simulink model "gate_V32_2016a_Sim"  (R2016a)
settings: Solver=FixedStepDiscrete  StartTime=0.0  StopTime=120  FixedStep=0.001  RelTol=1e-3
undefined symbols (not defined in the file): CLOSE_CHAR, CLOSE_SIDE_VALUE, CLOSED, CLOSING, CURRENT_STABLE_TIMER, CURRENT_THRESH, INIT, MOVING_TIMER, NO_PASS_ASSIG, OPEN, OPEN_CHAR, OPEN_SIDE_VALUE, OPEN_TIMEOUT, OPENING, OPENING_ACTIVE, PASS_ASSIGNED, PASS_INCOMPLETE, PASS_TIMEOUT, PASSWORD_VERIFIED, STABLE_TIMER_VALUE, TIMEOUT, WRONG_PASSWORD
(part 1 of 2)
settings Model: ExtModeTrigDuration=2  Creator=omaro  LastModifiedBy=oelkawok
settings DataIOCC: SaveFormat=StructureWithTime
settings OptimizationCC: DefaultParameterBehavior=Inlined  StateBitsets=on  DataBitsets=on  LifeSpan=1  MaxStackSize=64
settings DebuggingCC: ConsistencyChecking=error  ArrayBoundsChecking=error  SignalInfNanChecking=error  SignalRangeChecking=error  ReadBeforeWriteMsg=EnableAllAsError  WriteAfterWriteMsg=EnableAllAsError  WriteAfterReadMsg=EnableAllAsError  AlgebraicLoopMsg=error  ArtificialAlgebraicLoopMsg=error  BlockPriorityViolationMsg=error  MinStepSizeMsg=error  CheckMatrixSingularityMsg=error  ParameterUnderflowMsg=error  ParameterPrecisionLossMsg=error  UnderSpecifiedDataTypeMsg=warning  UnnecessaryDatatypeConvMsg=warning  VectorMatrixConversionMsg=error  SignalLabelMismatchMsg=error  UnconnectedInputMsg=error  UnconnectedOutputMsg=error  UnconnectedLineMsg=error  SFcnCompatibilityMsg=error  UniqueDataStoreMsg=error  BusObjectLabelMismatch=error  RootOutportRequireBusObject=error  ModelReferenceIOMsg=error  ModelReferenceVersionMismatchMessage=error  ModelReferenceIOMismatchMessage=error  ModelReferenceDataLoggingMessage=error  StrictBusMsg=ErrorOnBusTreatedAsVector  SFUnusedDataAndEventsDiag=error  SFUnexpectedBacktrackingDiag=error  SFInvalidInputDataAccessInChartInitDiag=error  SFNoUnconditionalDefaultTransitionDiag=error  SFTransitionOutsideNaturalParentDiag=error  SFUndirectedBroadcastEventsDiag=error  SFTransitionActionBeforeConditionDiag=error  SFOutputUsedAsStateInMooreChartDiag=warning
settings HardwareCC: ProdLongLongMode=on
settings SFSimCC: SimCustomHeaderCode=|
  | //#include "C:\Users\omaro\Desktop\Gate_Model\Arduino\Arduino.h"
  | //#include "Keypad\Keypad.h"
settings RTWCC: SystemTargetFile=ert.tlc  TemplateMakefile=ert_default_tmf  GenerateReport=on  RTWUseSimCustomCode=on  Toolchain=Arduino AVR v1.6.1  BuildConfiguration=Faster Runs  LaunchReport=on
settings RTWCC: CustomHeaderCode=|
  | //#include "C:\Users\omaro\Desktop\Gate_Model\Arduino\Arduino.h"
  | //#include "Keypad\Keypad.h"
settings CodeAppCC: ForceParamTrailComments=on  OperatorAnnotations=on  MATLABSourceComments=on
settings ERTTargetCC: ERTCustomFileBanners=off  SupportContinuousTime=on  SupportNonInlinedSFcns=on  SupportVariableSizeSignals=on  ModelStepFunctionPrototypeControlCompliant=off  RootIOFormat=Structure reference  ERTCustomFileTemplate=example_file_process.tlc

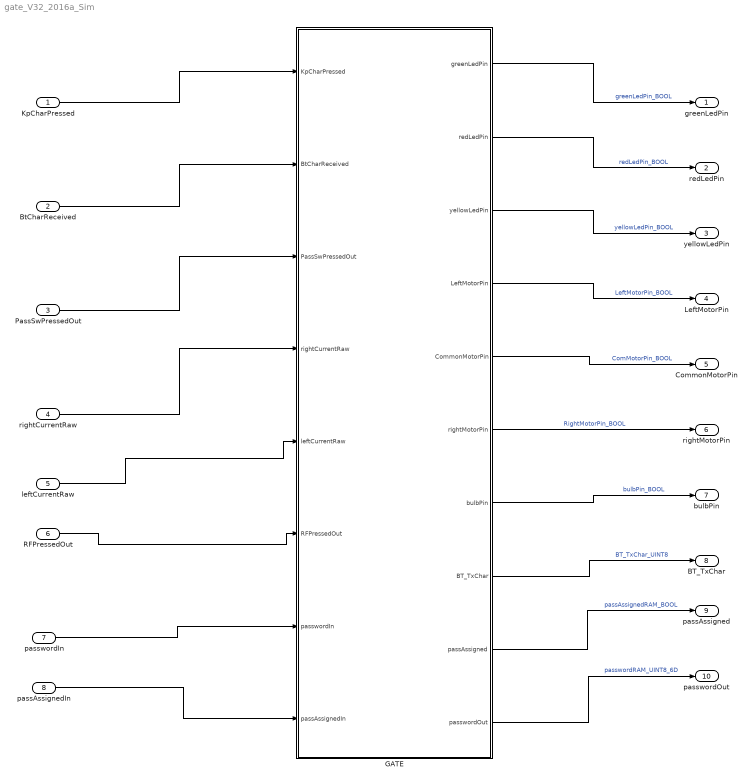
== system gate_V32_2016a_Sim ==
  "KpCharPressed " : Inport
  "BtCharReceived " : Inport  Port=2
  "PassSwPressedOut " : Inport  Port=3
  rightCurrentRaw : Inport  Port=4
  leftCurrentRaw : Inport  Port=5
  RFPressedOut : Inport  Port=6
  passwordIn : Inport  Port=7
  passAssignedIn : Inport  Port=8
  GATE : Subsystem  Variant=on  VariantControl=Variant1  OverrideUsingVariant=VariantB
  " greenLedPin" : Outport
  " redLedPin" : Outport  Port=2
  " yellowLedPin" : Outport  Port=3
  " LeftMotorPin" : Outport  Port=4
  " CommonMotorPin" : Outport  Port=5
  " rightMotorPin" : Outport  Port=6
  " bulbPin" : Outport  Port=7
  " BT_TxChar" : Outport  Port=8
  passAssigned : Outport  Port=9
  passwordOut : Outport  Port=10
  wires:
  passwordIn/1 -> GATE/7(passwordIn)
  "KpCharPressed "/1 -> GATE/1("KpCharPressed ")
  passAssignedIn/1 -> GATE/8(passAssignedIn)
  "BtCharReceived "/1 -> GATE/2("BtCharReceived ")
  leftCurrentRaw/1 -> GATE/5(leftCurrentRaw)
  "PassSwPressedOut "/1 -> GATE/3("PassSwPressedOut ")
  rightCurrentRaw/1 -> GATE/4(rightCurrentRaw)
  RFPressedOut/1 -> GATE/6(RFPressedOut)
  GATE/6(" rightMotorPin") -> " rightMotorPin"/1  "RightMotorPin_BOOL"
  GATE/5(" CommonMotorPin") -> " CommonMotorPin"/1  "ComMotorPin_BOOL"
  GATE/7(" bulbPin") -> " bulbPin"/1  "bulbPin_BOOL"
  GATE/4(" LeftMotorPin") -> " LeftMotorPin"/1  "LeftMotorPin_BOOL"
  GATE/8(" BT_TxChar") -> " BT_TxChar"/1  "BT_TxChar_UINT8"
  GATE/3(" yellowLedPin") -> " yellowLedPin"/1  "yellowLedPin_BOOL"
  GATE/2(" redLedPin") -> " redLedPin"/1  "redLedPin_BOOL"
  GATE/1(" greenLedPin") -> " greenLedPin"/1  "greenLedPin_BOOL"
  GATE/9(passAssigned) -> passAssigned/1  "passAssignedRAM_BOOL"
  GATE/10(passwordOut) -> passwordOut/1  "passwordRAM_UINT8_6D"

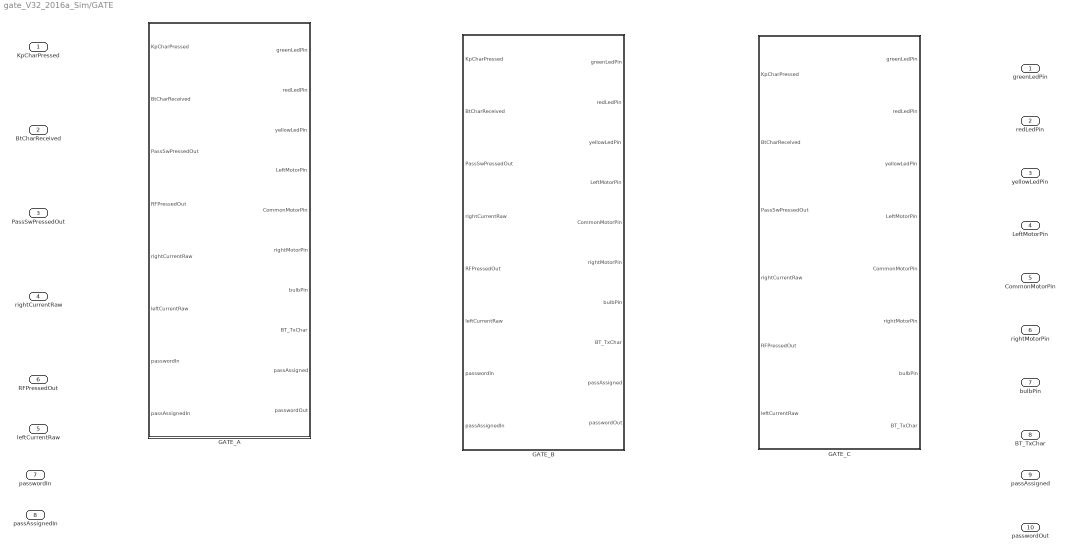
== system gate_V32_2016a_Sim/GATE ==
  "KpCharPressed " : Inport
  "BtCharReceived " : Inport  Port=2
  "PassSwPressedOut " : Inport  Port=3
  rightCurrentRaw : Inport  Port=4
  leftCurrentRaw : Inport  Port=5
  RFPressedOut : Inport  Port=6
  passwordIn : Inport  Port=7
  passAssignedIn : Inport  Port=8
  GATE_A : Subsystem  VariantControl=VariantA
  GATE_B : Subsystem  VariantControl=VariantB
  GATE_C : Subsystem  VariantControl=VariantC
  " greenLedPin" : Outport
  " redLedPin" : Outport  Port=2
  " yellowLedPin" : Outport  Port=3
  " LeftMotorPin" : Outport  Port=4
  " CommonMotorPin" : Outport  Port=5
  " rightMotorPin" : Outport  Port=6
  " bulbPin" : Outport  Port=7
  " BT_TxChar" : Outport  Port=8
  passAssigned : Outport  Port=9
  passwordOut : Outport  Port=10

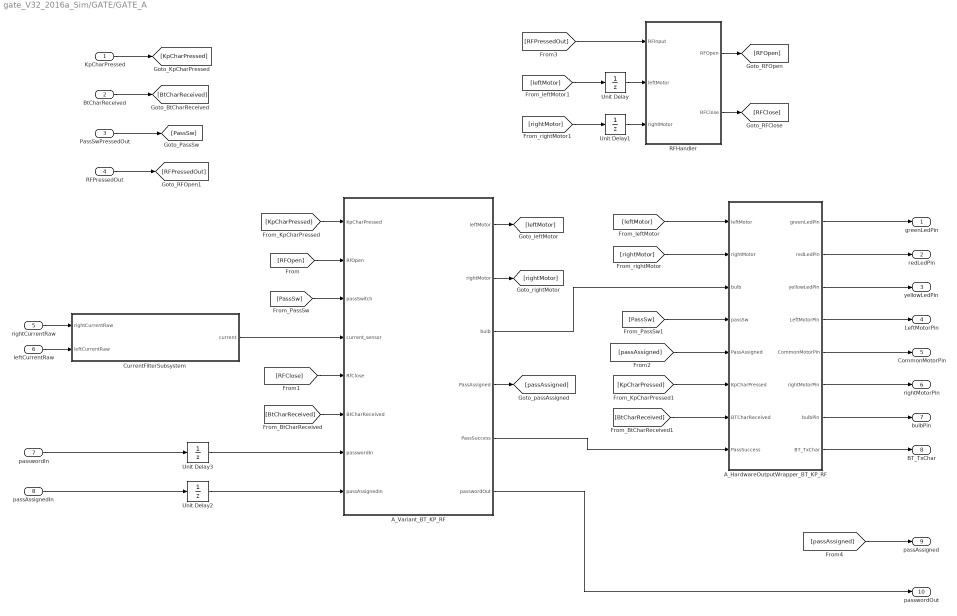
== system gate_V32_2016a_Sim/GATE/GATE_A ==
  KpCharPressed : Inport
  BtCharReceived : Inport  Port=2
  PassSwPressedOut : Inport  Port=3
  RFPressedOut : Inport  Port=4
  rightCurrentRaw : Inport  Port=5
  leftCurrentRaw : Inport  Port=6
  passwordIn : Inport  Port=7
  passAssignedIn : Inport  Port=8
  A_HardwareOutputWrapper_BT_KP_RF : Subsystem  VariantControl=Variant1
  A_Variant_BT_KP_RF : Subsystem  VariantControl=Variant
  CurrentFilterSubsystem : Subsystem
  RFHandler : Subsystem
  Unit Delay{,1..3} (4 alike) : UnitDelay  SampleTime=-1
  greenLedPin : Outport
  redLedPin : Outport  Port=2
  yellowLedPin : Outport  Port=3
  LeftMotorPin : Outport  Port=4
  CommonMotorPin : Outport  Port=5
  rightMotorPin : Outport  Port=6
  bulbPin : Outport  Port=7
  BT_TxChar : Outport  Port=8
  passAssigned : Outport  Port=9
  passwordOut : Outport  Port=10
  wires:
  RFHandler/1(RFOpen) -> [RFOpen]
  RFHandler/2(RFClose) -> [RFClose]
  [RFPressedOut] -> RFHandler/1(RFInput)
  RFPressedOut/1 -> [RFPressedOut]
  PassSwPressedOut/1 -> [PassSw]
  [leftMotor] -> Unit Delay/1
  Unit Delay/1 -> RFHandler/2(leftMotor)
  [rightMotor] -> Unit Delay1/1
  Unit Delay1/1 -> RFHandler/3(rightMotor)
  BtCharReceived/1 -> [BtCharReceived]
  KpCharPressed/1 -> [KpCharPressed]
  [RFOpen] -> A_Variant_BT_KP_RF/2(RfOpen)
  [PassSw] -> A_Variant_BT_KP_RF/3(passSwitch)
  [RFClose] -> A_Variant_BT_KP_RF/5(RfClose)
  [BtCharReceived] -> A_Variant_BT_KP_RF/6(BtCharReceived)
  A_Variant_BT_KP_RF/1(leftMotor) -> [leftMotor]
  A_Variant_BT_KP_RF/2(rightMotor) -> [rightMotor]
  [KpCharPressed] -> A_Variant_BT_KP_RF/1(KpCharPressed)
  [leftMotor] -> A_HardwareOutputWrapper_BT_KP_RF/1(leftMotor)
  [rightMotor] -> A_HardwareOutputWrapper_BT_KP_RF/2(rightMotor)
  A_Variant_BT_KP_RF/3(bulb) -> A_HardwareOutputWrapper_BT_KP_RF/3(bulb)
  [PassSw] -> A_HardwareOutputWrapper_BT_KP_RF/4(passSw)
  [KpCharPressed] -> A_HardwareOutputWrapper_BT_KP_RF/6(KpCharPressed)
  [BtCharReceived] -> A_HardwareOutputWrapper_BT_KP_RF/7(BTCharReceived)
  A_HardwareOutputWrapper_BT_KP_RF/1(greenLedPin) -> greenLedPin/1
  A_HardwareOutputWrapper_BT_KP_RF/2(redLedPin) -> redLedPin/1
  A_HardwareOutputWrapper_BT_KP_RF/3(yellowLedPin) -> yellowLedPin/1
  A_HardwareOutputWrapper_BT_KP_RF/4(LeftMotorPin) -> LeftMotorPin/1
  A_HardwareOutputWrapper_BT_KP_RF/5(CommonMotorPin) -> CommonMotorPin/1
  A_HardwareOutputWrapper_BT_KP_RF/6(rightMotorPin) -> rightMotorPin/1
  A_HardwareOutputWrapper_BT_KP_RF/7(bulbPin) -> bulbPin/1
  A_HardwareOutputWrapper_BT_KP_RF/8(BT_TxChar) -> BT_TxChar/1
  A_Variant_BT_KP_RF/4(PassAssigned) -> [passAssigned]
  [passAssigned] -> A_HardwareOutputWrapper_BT_KP_RF/5(PassAssigned)
  Unit Delay2/1 -> A_Variant_BT_KP_RF/8(passAssignedIn)
  Unit Delay3/1 -> A_Variant_BT_KP_RF/7(passwordIn)
  A_Variant_BT_KP_RF/5(PassSuccess) -> A_HardwareOutputWrapper_BT_KP_RF/8(PassSuccess)
  CurrentFilterSubsystem/1(current) -> A_Variant_BT_KP_RF/4(current_sensor)
  rightCurrentRaw/1 -> CurrentFilterSubsystem/1(rightCurrentRaw)
  leftCurrentRaw/1 -> CurrentFilterSubsystem/2(leftCurrentRaw)
  passAssignedIn/1 -> Unit Delay2/1
  passwordIn/1 -> Unit Delay3/1
  A_Variant_BT_KP_RF/6(passwordOut) -> passwordOut/1
  [passAssigned] -> passAssigned/1

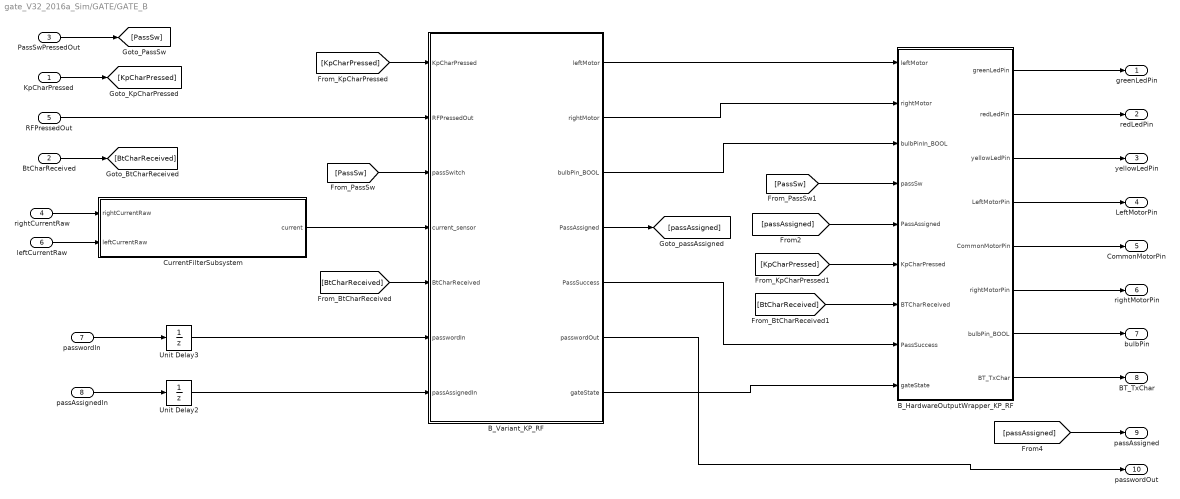
== system gate_V32_2016a_Sim/GATE/GATE_B ==
  KpCharPressed : Inport
  BtCharReceived : Inport  Port=2
  PassSwPressedOut : Inport  Port=3
  rightCurrentRaw : Inport  Port=4
  RFPressedOut : Inport  Port=5
  leftCurrentRaw : Inport  Port=6
  passwordIn : Inport  Port=7
  passAssignedIn : Inport  Port=8
  B_HardwareOutputWrapper_KP_RF : Subsystem  VariantControl=Variant2
  B_Variant_KP_RF : Subsystem  VariantControl=Variant2
  CurrentFilterSubsystem : Subsystem
  Unit Delay2 : UnitDelay  SampleTime=-1
  Unit Delay3 : UnitDelay  SampleTime=-1
  greenLedPin : Outport
  redLedPin : Outport  Port=2
  yellowLedPin : Outport  Port=3
  LeftMotorPin : Outport  Port=4
  CommonMotorPin : Outport  Port=5
  rightMotorPin : Outport  Port=6
  bulbPin : Outport  Port=7
  BT_TxChar : Outport  Port=8
  passAssigned : Outport  Port=9
  passwordOut : Outport  Port=10
  wires:
  CurrentFilterSubsystem/1(current) -> B_Variant_KP_RF/4(current_sensor)
  B_Variant_KP_RF/5(PassSuccess) -> B_HardwareOutputWrapper_KP_RF/8(PassSuccess)
  Unit Delay3/1 -> B_Variant_KP_RF/6(passwordIn)
  Unit Delay2/1 -> B_Variant_KP_RF/7(passAssignedIn)
  B_Variant_KP_RF/6(passwordOut) -> passwordOut/1
  [passAssigned] -> B_HardwareOutputWrapper_KP_RF/5(PassAssigned)
  B_Variant_KP_RF/4(PassAssigned) -> [passAssigned]
  B_HardwareOutputWrapper_KP_RF/8(BT_TxChar) -> BT_TxChar/1
  B_HardwareOutputWrapper_KP_RF/7(bulbPin_BOOL) -> bulbPin/1
  B_HardwareOutputWrapper_KP_RF/6(rightMotorPin) -> rightMotorPin/1
  B_HardwareOutputWrapper_KP_RF/5(CommonMotorPin) -> CommonMotorPin/1
  B_HardwareOutputWrapper_KP_RF/4(LeftMotorPin) -> LeftMotorPin/1
  B_HardwareOutputWrapper_KP_RF/3(yellowLedPin) -> yellowLedPin/1
  B_HardwareOutputWrapper_KP_RF/2(redLedPin) -> redLedPin/1
  B_HardwareOutputWrapper_KP_RF/1(greenLedPin) -> greenLedPin/1
  [BtCharReceived] -> B_HardwareOutputWrapper_KP_RF/7(BTCharReceived)
  [KpCharPressed] -> B_HardwareOutputWrapper_KP_RF/6(KpCharPressed)
  [PassSw] -> B_HardwareOutputWrapper_KP_RF/4(passSw)
  B_Variant_KP_RF/3(bulbPin_BOOL) -> B_HardwareOutputWrapper_KP_RF/3(bulbPinIn_BOOL)
  B_Variant_KP_RF/1(leftMotor) -> B_HardwareOutputWrapper_KP_RF/1(leftMotor)
  [KpCharPressed] -> B_Variant_KP_RF/1(KpCharPressed)
  [BtCharReceived] -> B_Variant_KP_RF/5(BtCharReceived)
  rightCurrentRaw/1 -> CurrentFilterSubsystem/1(rightCurrentRaw)
  [PassSw] -> B_Variant_KP_RF/3(passSwitch)
  RFPressedOut/1 -> B_Variant_KP_RF/2(RFPressedOut)
  KpCharPressed/1 -> [KpCharPressed]
  BtCharReceived/1 -> [BtCharReceived]
  PassSwPressedOut/1 -> [PassSw]
  leftCurrentRaw/1 -> CurrentFilterSubsystem/2(leftCurrentRaw)
  [passAssigned] -> passAssigned/1
  passAssignedIn/1 -> Unit Delay2/1
  passwordIn/1 -> Unit Delay3/1
  B_Variant_KP_RF/2(rightMotor) -> B_HardwareOutputWrapper_KP_RF/2(rightMotor)
  B_Variant_KP_RF/7(gateState) -> B_HardwareOutputWrapper_KP_RF/9(gateState)

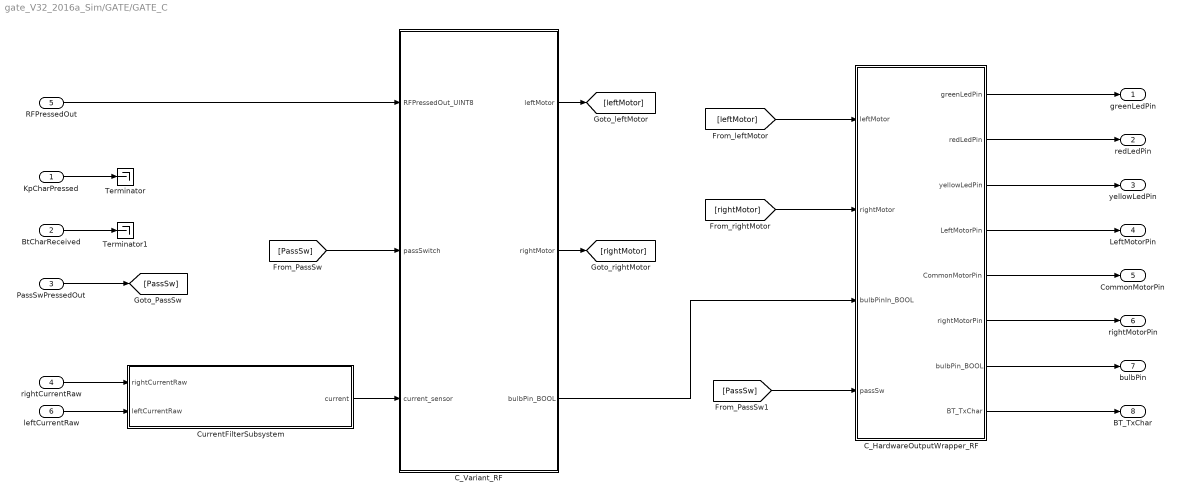
== system gate_V32_2016a_Sim/GATE/GATE_C ==
  KpCharPressed : Inport
  BtCharReceived : Inport  Port=2
  PassSwPressedOut : Inport  Port=3
  rightCurrentRaw : Inport  Port=4
  RFPressedOut : Inport  Port=5
  leftCurrentRaw : Inport  Port=6
  C_HardwareOutputWrapper_RF : Subsystem  VariantControl=Variant3
  C_Variant_RF : Subsystem  VariantControl=Variant3
  CurrentFilterSubsystem : Subsystem
  Terminator : Terminator
  Terminator1 : Terminator
  greenLedPin : Outport
  redLedPin : Outport  Port=2
  yellowLedPin : Outport  Port=3
  LeftMotorPin : Outport  Port=4
  CommonMotorPin : Outport  Port=5
  rightMotorPin : Outport  Port=6
  bulbPin : Outport  Port=7
  BT_TxChar : Outport  Port=8
  wires:
  PassSwPressedOut/1 -> [PassSw]
  BtCharReceived/1 -> Terminator1/1
  KpCharPressed/1 -> Terminator/1
  [PassSw] -> C_Variant_RF/2(passSwitch)
  rightCurrentRaw/1 -> CurrentFilterSubsystem/1(rightCurrentRaw)
  C_Variant_RF/1(leftMotor) -> [leftMotor]
  C_Variant_RF/2(rightMotor) -> [rightMotor]
  [leftMotor] -> C_HardwareOutputWrapper_RF/1(leftMotor)
  [rightMotor] -> C_HardwareOutputWrapper_RF/2(rightMotor)
  C_Variant_RF/3(bulbPin_BOOL) -> C_HardwareOutputWrapper_RF/3(bulbPinIn_BOOL)
  [PassSw] -> C_HardwareOutputWrapper_RF/4(passSw)
  C_HardwareOutputWrapper_RF/1(greenLedPin) -> greenLedPin/1
  C_HardwareOutputWrapper_RF/2(redLedPin) -> redLedPin/1
  C_HardwareOutputWrapper_RF/3(yellowLedPin) -> yellowLedPin/1
  C_HardwareOutputWrapper_RF/4(LeftMotorPin) -> LeftMotorPin/1
  C_HardwareOutputWrapper_RF/5(CommonMotorPin) -> CommonMotorPin/1
  C_HardwareOutputWrapper_RF/6(rightMotorPin) -> rightMotorPin/1
  C_HardwareOutputWrapper_RF/7(bulbPin_BOOL) -> bulbPin/1
  C_HardwareOutputWrapper_RF/8(BT_TxChar) -> BT_TxChar/1
  CurrentFilterSubsystem/1(current) -> C_Variant_RF/3(current_sensor)
  leftCurrentRaw/1 -> CurrentFilterSubsystem/2(leftCurrentRaw)
  RFPressedOut/1 -> C_Variant_RF/1(RFPressedOut_UINT8)

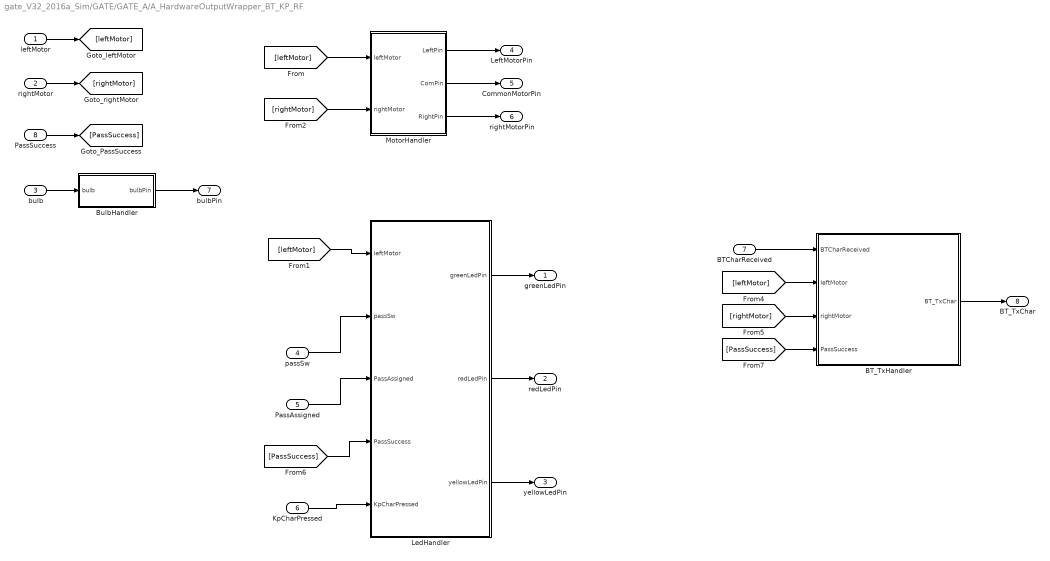
== system gate_V32_2016a_Sim/GATE/GATE_A/A_HardwareOutputWrapper_BT_KP_RF ==
  leftMotor : Inport
  rightMotor : Inport  Port=2
  bulb : Inport  Port=3
  passSw : Inport  Port=4
  PassAssigned : Inport  Port=5
  KpCharPressed : Inport  Port=6
  BTCharReceived : Inport  Port=7
  PassSuccess : Inport  Port=8
  BT_TxHandler : Subsystem
  BulbHandler : Subsystem
  LedHandler : Subsystem
  MotorHandler : Subsystem
  greenLedPin : Outport
  redLedPin : Outport  Port=2
  yellowLedPin : Outport  Port=3
  LeftMotorPin : Outport  Port=4
  CommonMotorPin : Outport  Port=5
  rightMotorPin : Outport  Port=6
  bulbPin : Outport  Port=7
  BT_TxChar : Outport  Port=8
  wires:
  [leftMotor] -> MotorHandler/1(leftMotor)
  [rightMotor] -> MotorHandler/2(rightMotor)
  bulb/1 -> BulbHandler/1(bulb)
  LedHandler/1(greenLedPin) -> greenLedPin/1
  LedHandler/2(redLedPin) -> redLedPin/1
  LedHandler/3(yellowLedPin) -> yellowLedPin/1
  MotorHandler/1(LeftPin) -> LeftMotorPin/1
  MotorHandler/2(ComPin) -> CommonMotorPin/1
  MotorHandler/3(RightPin) -> rightMotorPin/1
  BulbHandler/1(bulbPin) -> bulbPin/1
  leftMotor/1 -> [leftMotor]
  [leftMotor] -> LedHandler/1(leftMotor)
  rightMotor/1 -> [rightMotor]
  passSw/1 -> LedHandler/2(passSw)
  PassAssigned/1 -> LedHandler/3(PassAssigned)
  [PassSuccess] -> LedHandler/4(PassSuccess)
  KpCharPressed/1 -> LedHandler/5(KpCharPressed)
  [leftMotor] -> BT_TxHandler/2(leftMotor)
  BTCharReceived/1 -> BT_TxHandler/1(BTCharReceived)
  [rightMotor] -> BT_TxHandler/3(rightMotor)
  PassSuccess/1 -> [PassSuccess]
  [PassSuccess] -> BT_TxHandler/4(PassSuccess)
  BT_TxHandler/1(BT_TxChar) -> BT_TxChar/1

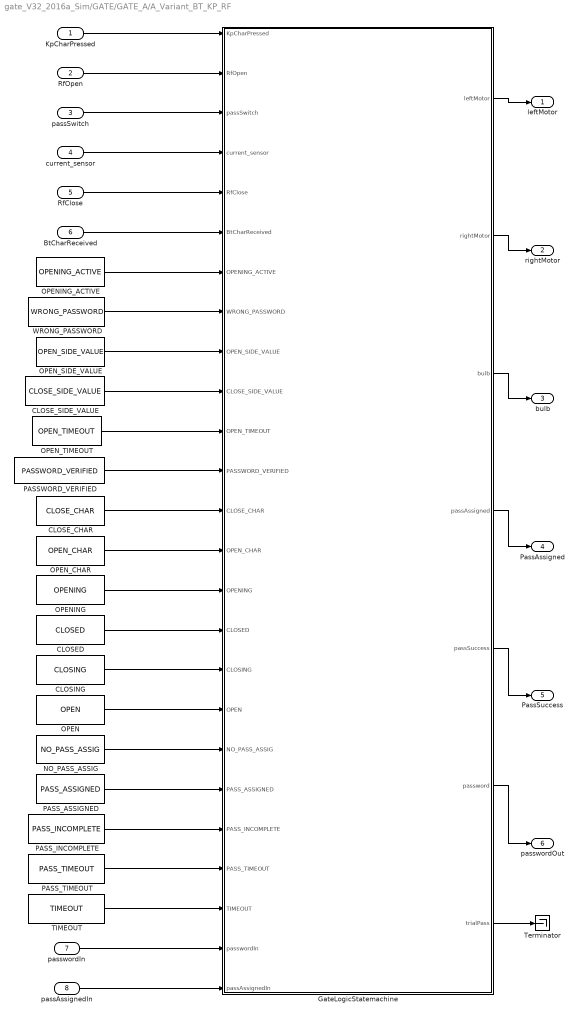
== system gate_V32_2016a_Sim/GATE/GATE_A/A_Variant_BT_KP_RF ==
  KpCharPressed : Inport
  RfOpen : Inport  Port=2
  passSwitch : Inport  Port=3
  current_sensor : Inport  Port=4
  RfClose : Inport  Port=5
  BtCharReceived : Inport  Port=6
  passwordIn : Inport  Port=7
  passAssignedIn : Inport  Port=8
  CLOSED : Constant  Value=CLOSED  SampleTime=-1
  CLOSE_CHAR : Constant  Value=CLOSE_CHAR  SampleTime=-1
  CLOSE_SIDE_VALUE : Constant  Value=CLOSE_SIDE_VALUE  SampleTime=-1
  CLOSING : Constant  Value=CLOSING  SampleTime=-1
  GateLogicStatemachine : Stateflow chart  TreatAsAtomicUnit=on
  NO_PASS_ASSIG : Constant  Value=NO_PASS_ASSIG  SampleTime=-1
  OPEN : Constant  Value=OPEN  SampleTime=-1
  OPENING : Constant  Value=OPENING  SampleTime=-1
  OPENING_ACTIVE : Constant  Value=OPENING_ACTIVE  SampleTime=-1
  OPEN_CHAR : Constant  Value=OPEN_CHAR  SampleTime=-1
  OPEN_SIDE_VALUE : Constant  Value=OPEN_SIDE_VALUE  SampleTime=-1
  OPEN_TIMEOUT : Constant  Value=OPEN_TIMEOUT  SampleTime=-1
  PASSWORD_VERIFIED : Constant  Value=PASSWORD_VERIFIED  SampleTime=-1
  PASS_ASSIGNED : Constant  Value=PASS_ASSIGNED  SampleTime=-1
  PASS_INCOMPLETE : Constant  Value=PASS_INCOMPLETE  SampleTime=-1
  PASS_TIMEOUT : Constant  Value=PASS_TIMEOUT  SampleTime=-1
  TIMEOUT : Constant  Value=TIMEOUT  SampleTime=-1
  Terminator : Terminator
  WRONG_PASSWORD : Constant  Value=WRONG_PASSWORD  SampleTime=-1
  leftMotor : Outport
  rightMotor : Outport  Port=2
  bulb : Outport  Port=3
  PassAssigned : Outport  Port=4
  PassSuccess : Outport  Port=5
  passwordOut : Outport  Port=6
  wires:
  RfClose/1 -> GateLogicStatemachine/5(RfClose)
  TIMEOUT/1 -> GateLogicStatemachine/23(TIMEOUT)
  PASS_INCOMPLETE/1 -> GateLogicStatemachine/21(PASS_INCOMPLETE)
  PASS_ASSIGNED/1 -> GateLogicStatemachine/20(PASS_ASSIGNED)
  GateLogicStatemachine/4(passAssigned) -> PassAssigned/1
  passSwitch/1 -> GateLogicStatemachine/3(passSwitch)
  GateLogicStatemachine/5(passSuccess) -> PassSuccess/1
  PASS_TIMEOUT/1 -> GateLogicStatemachine/22(PASS_TIMEOUT)
  KpCharPressed/1 -> GateLogicStatemachine/1(KpCharPressed)
  BtCharReceived/1 -> GateLogicStatemachine/6(BtCharReceived)
  NO_PASS_ASSIG/1 -> GateLogicStatemachine/19(NO_PASS_ASSIG)
  CLOSE_SIDE_VALUE/1 -> GateLogicStatemachine/10(CLOSE_SIDE_VALUE)
  OPEN_TIMEOUT/1 -> GateLogicStatemachine/11(OPEN_TIMEOUT)
  OPEN_SIDE_VALUE/1 -> GateLogicStatemachine/9(OPEN_SIDE_VALUE)
  OPENING_ACTIVE/1 -> GateLogicStatemachine/7(OPENING_ACTIVE)
  GateLogicStatemachine/2(rightMotor) -> rightMotor/1
  GateLogicStatemachine/1(leftMotor) -> leftMotor/1
  WRONG_PASSWORD/1 -> GateLogicStatemachine/8(WRONG_PASSWORD)
  current_sensor/1 -> GateLogicStatemachine/4(current_sensor)
  GateLogicStatemachine/3(bulb) -> bulb/1
  RfOpen/1 -> GateLogicStatemachine/2(RfOpen)
  PASSWORD_VERIFIED/1 -> GateLogicStatemachine/12(PASSWORD_VERIFIED)
  OPEN/1 -> GateLogicStatemachine/18(OPEN)
  CLOSE_CHAR/1 -> GateLogicStatemachine/13(CLOSE_CHAR)
  OPEN_CHAR/1 -> GateLogicStatemachine/14(OPEN_CHAR)
  CLOSED/1 -> GateLogicStatemachine/16(CLOSED)
  OPENING/1 -> GateLogicStatemachine/15(OPENING)
  CLOSING/1 -> GateLogicStatemachine/17(CLOSING)
  GateLogicStatemachine/6(password) -> passwordOut/1
  passwordIn/1 -> GateLogicStatemachine/24(passwordIn)
  passAssignedIn/1 -> GateLogicStatemachine/25(passAssignedIn)
  GateLogicStatemachine/7(trialPass) -> Terminator/1

== system gate_V32_2016a_Sim/GATE/GATE_A/CurrentFilterSubsystem ==
  rightCurrentRaw : Inport
  leftCurrentRaw : Inport  Port=2
  10msSmapler : Stateflow chart  TreatAsAtomicUnit=on
  Subsystem : Subsystem
  current : Outport
  wires:
  10msSmapler/1(triggerOn()) -> Subsystem/Trigger
  Subsystem/1(current) -> current/1
  rightCurrentRaw/1 -> Subsystem/1(rightCurrentRaw)
  leftCurrentRaw/1 -> Subsystem/2(leftCurrentRaw)

== system gate_V32_2016a_Sim/GATE/GATE_A/RFHandler ==
  RFInput : Inport
  leftMotor : Inport  Port=2
  rightMotor : Inport  Port=3
  CLOSED : Constant  Value=CLOSED  SampleTime=-1
  CLOSING : Constant  Value=CLOSING  SampleTime=-1
  OPEN : Constant  Value=OPEN  SampleTime=-1
  OPENING : Constant  Value=OPENING  SampleTime=-1
  RFHandlerL : Stateflow chart  TreatAsAtomicUnit=on
  RFOpen : Outport
  RFClose : Outport  Port=2
  wires:
  RFInput/1 -> RFHandlerL/1(btn)
  RFHandlerL/1(RFClose) -> RFClose/1
  RFHandlerL/2(RFOpen) -> RFOpen/1
  OPEN/1 -> RFHandlerL/6(OPEN)
  CLOSING/1 -> RFHandlerL/5(CLOSING)
  CLOSED/1 -> RFHandlerL/4(CLOSED)
  OPENING/1 -> RFHandlerL/7(OPENING)
  leftMotor/1 -> RFHandlerL/2(leftMotor)
  rightMotor/1 -> RFHandlerL/3(rightMotor)

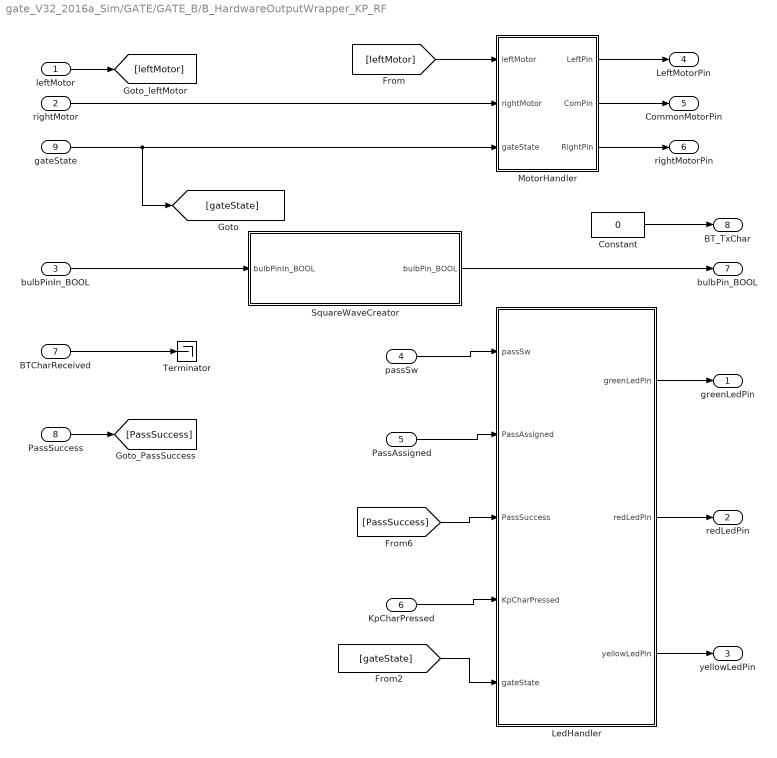
== system gate_V32_2016a_Sim/GATE/GATE_B/B_HardwareOutputWrapper_KP_RF ==
  leftMotor : Inport
  rightMotor : Inport  Port=2
  bulbPinIn_BOOL : Inport  Port=3
  passSw : Inport  Port=4
  PassAssigned : Inport  Port=5
  KpCharPressed : Inport  Port=6
  BTCharReceived : Inport  Port=7
  PassSuccess : Inport  Port=8
  gateState : Inport  Port=9
  Constant : Constant  Value=0  SampleTime=-1
  LedHandler : Subsystem
  MotorHandler : Subsystem
  SquareWaveCreator : Subsystem
  Terminator : Terminator
  greenLedPin : Outport
  redLedPin : Outport  Port=2
  yellowLedPin : Outport  Port=3
  LeftMotorPin : Outport  Port=4
  CommonMotorPin : Outport  Port=5
  rightMotorPin : Outport  Port=6
  bulbPin_BOOL : Outport  Port=7
  BT_TxChar : Outport  Port=8
  wires:
  rightMotor/1 -> MotorHandler/2(rightMotor)
  BTCharReceived/1 -> Terminator/1
  [leftMotor] -> MotorHandler/1(leftMotor)
  LedHandler/1(greenLedPin) -> greenLedPin/1
  LedHandler/2(redLedPin) -> redLedPin/1
  LedHandler/3(yellowLedPin) -> yellowLedPin/1
  MotorHandler/1(LeftPin) -> LeftMotorPin/1
  MotorHandler/2(ComPin) -> CommonMotorPin/1
  MotorHandler/3(RightPin) -> rightMotorPin/1
  bulbPinIn_BOOL/1 -> SquareWaveCreator/1(bulbPinIn_BOOL)
  leftMotor/1 -> [leftMotor]
  passSw/1 -> LedHandler/1(passSw)
  PassAssigned/1 -> LedHandler/2(PassAssigned)
  [PassSuccess] -> LedHandler/3(PassSuccess)
  KpCharPressed/1 -> LedHandler/4(KpCharPressed)
  PassSuccess/1 -> [PassSuccess]
  Constant/1 -> BT_TxChar/1
  gateState/1 -> [gateState], MotorHandler/3(gateState)
  SquareWaveCreator/1(bulbPin_BOOL) -> bulbPin_BOOL/1
  [gateState] -> LedHandler/5(gateState)

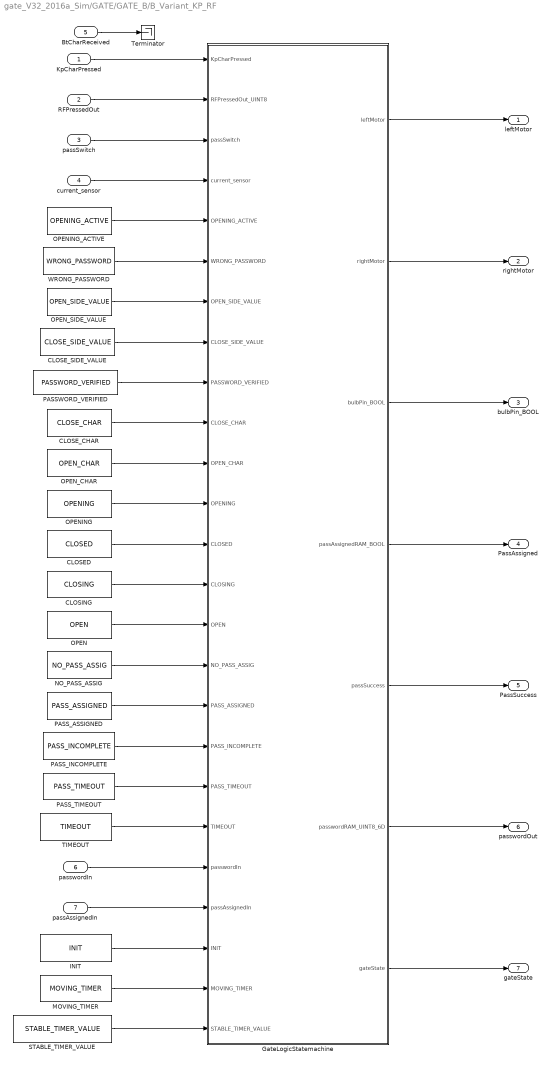
== system gate_V32_2016a_Sim/GATE/GATE_B/B_Variant_KP_RF ==
  KpCharPressed : Inport
  RFPressedOut : Inport  Port=2
  passSwitch : Inport  Port=3
  current_sensor : Inport  Port=4
  BtCharReceived : Inport  Port=5
  passwordIn : Inport  Port=6
  passAssignedIn : Inport  Port=7
  CLOSED : Constant  Value=CLOSED  SampleTime=-1
  CLOSE_CHAR : Constant  Value=CLOSE_CHAR  SampleTime=-1
  CLOSE_SIDE_VALUE : Constant  Value=CLOSE_SIDE_VALUE  SampleTime=-1
  CLOSING : Constant  Value=CLOSING  SampleTime=-1
  GateLogicStatemachine : Stateflow chart  TreatAsAtomicUnit=on
  INIT : Constant  Value=INIT  SampleTime=-1
  MOVING_TIMER : Constant  Value=MOVING_TIMER  SampleTime=-1
  NO_PASS_ASSIG : Constant  Value=NO_PASS_ASSIG  SampleTime=-1
  OPEN : Constant  Value=OPEN  SampleTime=-1
  OPENING : Constant  Value=OPENING  SampleTime=-1
  OPENING_ACTIVE : Constant  Value=OPENING_ACTIVE  SampleTime=-1
  OPEN_CHAR : Constant  Value=OPEN_CHAR  SampleTime=-1
  OPEN_SIDE_VALUE : Constant  Value=OPEN_SIDE_VALUE  SampleTime=-1
  PASSWORD_VERIFIED : Constant  Value=PASSWORD_VERIFIED  SampleTime=-1
  PASS_ASSIGNED : Constant  Value=PASS_ASSIGNED  SampleTime=-1
  PASS_INCOMPLETE : Constant  Value=PASS_INCOMPLETE  SampleTime=-1
  PASS_TIMEOUT : Constant  Value=PASS_TIMEOUT  SampleTime=-1
  STABLE_TIMER_VALUE : Constant  Value=STABLE_TIMER_VALUE  SampleTime=-1
  TIMEOUT : Constant  Value=TIMEOUT  SampleTime=-1
  Terminator : Terminator
  WRONG_PASSWORD : Constant  Value=WRONG_PASSWORD  SampleTime=-1
  leftMotor : Outport
  rightMotor : Outport  Port=2
  bulbPin_BOOL : Outport  Port=3
  PassAssigned : Outport  Port=4
  PassSuccess : Outport  Port=5
  passwordOut : Outport  Port=6
  gateState : Outport  Port=7
  wires:
  GateLogicStatemachine/6(passwordRAM_UINT8_6D) -> passwordOut/1
  passAssignedIn/1 -> GateLogicStatemachine/22(passAssignedIn)
  passwordIn/1 -> GateLogicStatemachine/21(passwordIn)
  BtCharReceived/1 -> Terminator/1
  TIMEOUT/1 -> GateLogicStatemachine/20(TIMEOUT)
  PASS_INCOMPLETE/1 -> GateLogicStatemachine/18(PASS_INCOMPLETE)
  PASS_ASSIGNED/1 -> GateLogicStatemachine/17(PASS_ASSIGNED)
  GateLogicStatemachine/4(passAssignedRAM_BOOL) -> PassAssigned/1
  passSwitch/1 -> GateLogicStatemachine/3(passSwitch)
  GateLogicStatemachine/5(passSuccess) -> PassSuccess/1
  PASS_TIMEOUT/1 -> GateLogicStatemachine/19(PASS_TIMEOUT)
  KpCharPressed/1 -> GateLogicStatemachine/1(KpCharPressed)
  NO_PASS_ASSIG/1 -> GateLogicStatemachine/16(NO_PASS_ASSIG)
  CLOSE_SIDE_VALUE/1 -> GateLogicStatemachine/8(CLOSE_SIDE_VALUE)
  OPEN_SIDE_VALUE/1 -> GateLogicStatemachine/7(OPEN_SIDE_VALUE)
  OPENING_ACTIVE/1 -> GateLogicStatemachine/5(OPENING_ACTIVE)
  GateLogicStatemachine/2(rightMotor) -> rightMotor/1
  GateLogicStatemachine/1(leftMotor) -> leftMotor/1
  WRONG_PASSWORD/1 -> GateLogicStatemachine/6(WRONG_PASSWORD)
  current_sensor/1 -> GateLogicStatemachine/4(current_sensor)
  GateLogicStatemachine/3(bulbPin_BOOL) -> bulbPin_BOOL/1
  RFPressedOut/1 -> GateLogicStatemachine/2(RFPressedOut_UINT8)
  PASSWORD_VERIFIED/1 -> GateLogicStatemachine/9(PASSWORD_VERIFIED)
  OPEN/1 -> GateLogicStatemachine/15(OPEN)
  CLOSE_CHAR/1 -> GateLogicStatemachine/10(CLOSE_CHAR)
  OPEN_CHAR/1 -> GateLogicStatemachine/11(OPEN_CHAR)
  CLOSED/1 -> GateLogicStatemachine/13(CLOSED)
  OPENING/1 -> GateLogicStatemachine/12(OPENING)
  CLOSING/1 -> GateLogicStatemachine/14(CLOSING)
  GateLogicStatemachine/7(gateState) -> gateState/1
  INIT/1 -> GateLogicStatemachine/23(INIT)
  MOVING_TIMER/1 -> GateLogicStatemachine/24(MOVING_TIMER)
  STABLE_TIMER_VALUE/1 -> GateLogicStatemachine/25(STABLE_TIMER_VALUE)

== system gate_V32_2016a_Sim/GATE/GATE_B/CurrentFilterSubsystem ==
  rightCurrentRaw : Inport
  leftCurrentRaw : Inport  Port=2
  10msSmapler : Stateflow chart  Commented=on  TreatAsAtomicUnit=on
  Subsystem : Subsystem
  current : Outport
  wires:
  Subsystem/1(current) -> current/1
  rightCurrentRaw/1 -> Subsystem/1(rightCurrentRaw)
  leftCurrentRaw/1 -> Subsystem/2(leftCurrentRaw)

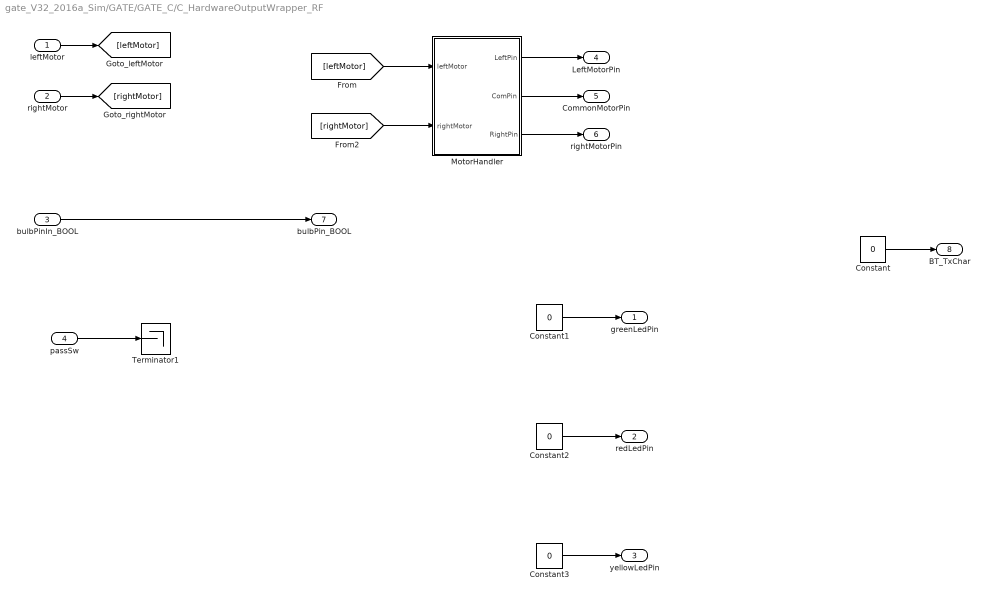
== system gate_V32_2016a_Sim/GATE/GATE_C/C_HardwareOutputWrapper_RF ==
  leftMotor : Inport
  rightMotor : Inport  Port=2
  bulbPinIn_BOOL : Inport  Port=3
  passSw : Inport  Port=4
  Constant{,1..3} (4 alike) : Constant  Value=0  SampleTime=-1
  MotorHandler : Subsystem
  Terminator1 : Terminator
  greenLedPin : Outport
  redLedPin : Outport  Port=2
  yellowLedPin : Outport  Port=3
  LeftMotorPin : Outport  Port=4
  CommonMotorPin : Outport  Port=5
  rightMotorPin : Outport  Port=6
  bulbPin_BOOL : Outport  Port=7
  BT_TxChar : Outport  Port=8
  wires:
  [leftMotor] -> MotorHandler/1(leftMotor)
  [rightMotor] -> MotorHandler/2(rightMotor)
  MotorHandler/1(LeftPin) -> LeftMotorPin/1
  MotorHandler/2(ComPin) -> CommonMotorPin/1
  MotorHandler/3(RightPin) -> rightMotorPin/1
  bulbPinIn_BOOL/1 -> bulbPin_BOOL/1
  leftMotor/1 -> [leftMotor]
  rightMotor/1 -> [rightMotor]
  Constant/1 -> BT_TxChar/1
  Constant3/1 -> yellowLedPin/1
  Constant2/1 -> redLedPin/1
  Constant1/1 -> greenLedPin/1
  passSw/1 -> Terminator1/1

== system gate_V32_2016a_Sim/GATE/GATE_C/C_Variant_RF ==
  RFPressedOut_UINT8 : Inport
  passSwitch : Inport  Port=2
  current_sensor : Inport  Port=3
  CLOSED : Constant  Value=CLOSED  SampleTime=-1
  CLOSE_SIDE_VALUE : Constant  Value=CLOSE_SIDE_VALUE  SampleTime=-1
  CLOSING : Constant  Value=CLOSING  SampleTime=-1
  GateLogicStatemachine : Stateflow chart  TreatAsAtomicUnit=on
  OPEN : Constant  Value=OPEN  SampleTime=-1
  OPENING : Constant  Value=OPENING  SampleTime=-1
  OPENING_ACTIVE : Constant  Value=OPENING_ACTIVE  SampleTime=-1
  OPEN_SIDE_VALUE : Constant  Value=OPEN_SIDE_VALUE  SampleTime=-1
  leftMotor : Outport
  rightMotor : Outport  Port=2
  bulbPin_BOOL : Outport  Port=3
  wires:
  passSwitch/1 -> GateLogicStatemachine/2(passSwitch)
  CLOSE_SIDE_VALUE/1 -> GateLogicStatemachine/6(CLOSE_SIDE_VALUE)
  OPEN_SIDE_VALUE/1 -> GateLogicStatemachine/5(OPEN_SIDE_VALUE)
  OPENING_ACTIVE/1 -> GateLogicStatemachine/4(OPENING_ACTIVE)
  GateLogicStatemachine/2(rightMotor) -> rightMotor/1
  GateLogicStatemachine/1(leftMotor) -> leftMotor/1
  current_sensor/1 -> GateLogicStatemachine/3(current_sensor)
  GateLogicStatemachine/3(bulbPin_BOOL) -> bulbPin_BOOL/1
  RFPressedOut_UINT8/1 -> GateLogicStatemachine/1(RFPressedOut_UINT8)
  OPEN/1 -> GateLogicStatemachine/10(OPEN)
  CLOSED/1 -> GateLogicStatemachine/8(CLOSED)
  OPENING/1 -> GateLogicStatemachine/7(OPENING)
  CLOSING/1 -> GateLogicStatemachine/9(CLOSING)

== system gate_V32_2016a_Sim/GATE/GATE_C/CurrentFilterSubsystem ==
  rightCurrentRaw : Inport
  leftCurrentRaw : Inport  Port=2
  10msSmapler : Stateflow chart  TreatAsAtomicUnit=on
  Subsystem : Subsystem
  current : Outport
  wires:
  rightCurrentRaw/1 -> Subsystem/1(rightCurrentRaw)
  Subsystem/1(current) -> current/1
  10msSmapler/1(triggerOn()) -> Subsystem/Trigger
  leftCurrentRaw/1 -> Subsystem/2(leftCurrentRaw)

== system gate_V32_2016a_Sim/GATE/GATE_A/A_HardwareOutputWrapper_BT_KP_RF/BT_TxHandler ==
  BTCharReceived : Inport
  leftMotor : Inport  Port=2
  rightMotor : Inport  Port=3
  PassSuccess : Inport  Port=4
  BT_TxHandler : Stateflow chart  TreatAsAtomicUnit=on
  CLOSED : Constant  Value=CLOSED  SampleTime=-1
  CLOSING : Constant  Value=CLOSING  SampleTime=-1
  OPEN : Constant  Value=OPEN  SampleTime=-1
  OPENING : Constant  Value=OPENING  SampleTime=-1
  WRONG_PASSWORD : Constant  Value=WRONG_PASSWORD  SampleTime=-1
  BT_TxChar : Outport
  wires:
  BTCharReceived/1 -> BT_TxHandler/1(BTCharReceived)
  leftMotor/1 -> BT_TxHandler/2(leftMotor)
  rightMotor/1 -> BT_TxHandler/3(rightMotor)
  BT_TxHandler/1(BT_TxChar) -> BT_TxChar/1
  PassSuccess/1 -> BT_TxHandler/4(PassSuccess)
  CLOSED/1 -> BT_TxHandler/5(CLOSED)
  CLOSING/1 -> BT_TxHandler/6(CLOSING)
  OPEN/1 -> BT_TxHandler/7(OPEN)
  OPENING/1 -> BT_TxHandler/8(OPENING)
  WRONG_PASSWORD/1 -> BT_TxHandler/9(WRONG_PASSWORD)

== system gate_V32_2016a_Sim/GATE/GATE_A/A_HardwareOutputWrapper_BT_KP_RF/BulbHandler ==
  bulb : Inport
  bulbPin : Outport
  wires:
  bulb/1 -> bulbPin/1

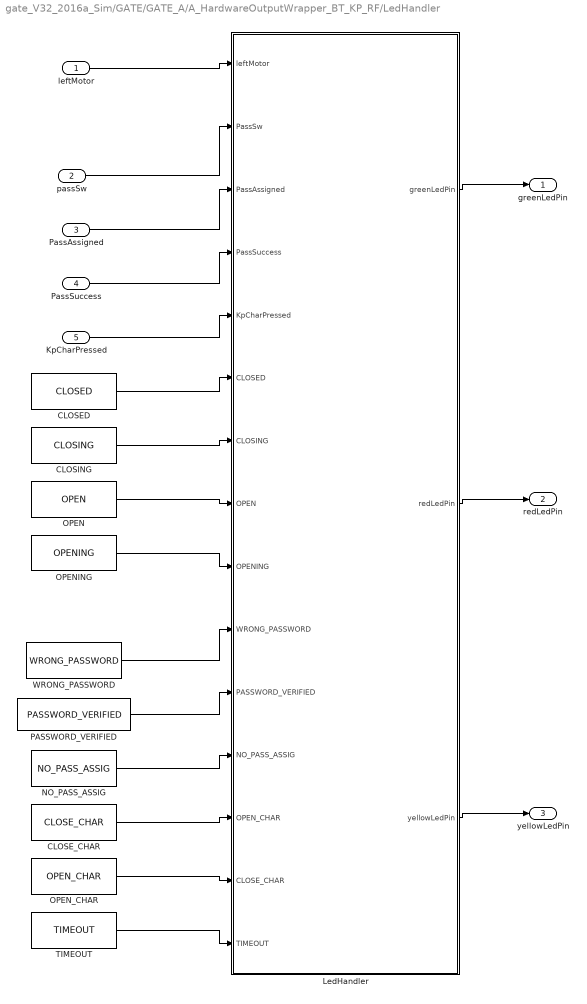
== system gate_V32_2016a_Sim/GATE/GATE_A/A_HardwareOutputWrapper_BT_KP_RF/LedHandler ==
  leftMotor : Inport
  passSw : Inport  Port=2
  PassAssigned : Inport  Port=3
  PassSuccess : Inport  Port=4
  KpCharPressed : Inport  Port=5
  CLOSED : Constant  Value=CLOSED  SampleTime=-1
  CLOSE_CHAR : Constant  Value=CLOSE_CHAR  SampleTime=-1
  CLOSING : Constant  Value=CLOSING  SampleTime=-1
  LedHandler : Stateflow chart  TreatAsAtomicUnit=on
  NO_PASS_ASSIG : Constant  Value=NO_PASS_ASSIG  SampleTime=-1
  OPEN : Constant  Value=OPEN  SampleTime=-1
  OPENING : Constant  Value=OPENING  SampleTime=-1
  OPEN_CHAR : Constant  Value=OPEN_CHAR  SampleTime=-1
  PASSWORD_VERIFIED : Constant  Value=PASSWORD_VERIFIED  SampleTime=-1
  TIMEOUT : Constant  Value=TIMEOUT  SampleTime=-1
  WRONG_PASSWORD : Constant  Value=WRONG_PASSWORD  SampleTime=-1
  greenLedPin : Outport
  redLedPin : Outport  Port=2
  yellowLedPin : Outport  Port=3
  wires:
  leftMotor/1 -> LedHandler/1(leftMotor)
  LedHandler/1(greenLedPin) -> greenLedPin/1
  LedHandler/2(redLedPin) -> redLedPin/1
  LedHandler/3(yellowLedPin) -> yellowLedPin/1
  passSw/1 -> LedHandler/2(PassSw)
  PassAssigned/1 -> LedHandler/3(PassAssigned)
  PassSuccess/1 -> LedHandler/4(PassSuccess)
  OPENING/1 -> LedHandler/9(OPENING)
  OPEN/1 -> LedHandler/8(OPEN)
  CLOSING/1 -> LedHandler/7(CLOSING)
  CLOSED/1 -> LedHandler/6(CLOSED)
  WRONG_PASSWORD/1 -> LedHandler/10(WRONG_PASSWORD)
  PASSWORD_VERIFIED/1 -> LedHandler/11(PASSWORD_VERIFIED)
  NO_PASS_ASSIG/1 -> LedHandler/12(NO_PASS_ASSIG)
  KpCharPressed/1 -> LedHandler/5(KpCharPressed)
  CLOSE_CHAR/1 -> LedHandler/13(OPEN_CHAR)
  OPEN_CHAR/1 -> LedHandler/14(CLOSE_CHAR)
  TIMEOUT/1 -> LedHandler/15(TIMEOUT)

== system gate_V32_2016a_Sim/GATE/GATE_A/A_HardwareOutputWrapper_BT_KP_RF/MotorHandler ==
  leftMotor : Inport
  rightMotor : Inport  Port=2
  CLOSED : Constant  Value=CLOSED  SampleTime=-1
  CLOSING : Constant  Value=CLOSING  SampleTime=-1
  MotorsHandler : Stateflow chart  TreatAsAtomicUnit=on
  OPEN : Constant  Value=OPEN  SampleTime=-1
  OPENING : Constant  Value=OPENING  SampleTime=-1
  Unit Delay : UnitDelay  SampleTime=-1
  Unit Delay1 : UnitDelay  SampleTime=-1
  LeftPin : Outport
  ComPin : Outport  Port=2
  RightPin : Outport  Port=3
  wires:
  leftMotor/1 -> Unit Delay/1, MotorsHandler/1(leftMotor)
  Unit Delay/1 -> MotorsHandler/2(oldLeft)
  rightMotor/1 -> Unit Delay1/1, MotorsHandler/3(rightMotor)
  Unit Delay1/1 -> MotorsHandler/4(oldRight)
  CLOSED/1 -> MotorsHandler/5(CLOSED)
  CLOSING/1 -> MotorsHandler/6(CLOSING)
  OPEN/1 -> MotorsHandler/7(OPEN)
  OPENING/1 -> MotorsHandler/8(OPENING)
  MotorsHandler/1(LeftPin) -> LeftPin/1
  MotorsHandler/2(ComPin) -> ComPin/1
  MotorsHandler/3(RightPin) -> RightPin/1

== system gate_V32_2016a_Sim/GATE/GATE_A/CurrentFilterSubsystem/Subsystem ==
  rightCurrentRaw : Inport
  leftCurrentRaw : Inport  Port=2
  Trigger : TriggerPort  TriggerType=function-call  VariantControl=Variant  PortDimensions=1
  Logical Operator : Logic  Operator=OR  AllPortsSameDT=off  OutDataTypeStr=boolean
  SquareWaveDetector : Stateflow chart  TreatAsAtomicUnit=on
  SquareWaveDetector1 : Stateflow chart  TreatAsAtomicUnit=on
  Unit Delay : UnitDelay  SampleTime=-1
  Unit Delay1 : UnitDelay  SampleTime=-1
  current : Outport
  wires:
  rightCurrentRaw/1 -> SquareWaveDetector/1(CurrentAnalogIn), Unit Delay/1
  Unit Delay/1 -> SquareWaveDetector/2(CurrentAnalogInOld)
  leftCurrentRaw/1 -> Unit Delay1/1, SquareWaveDetector1/1(CurrentAnalogIn)
  Unit Delay1/1 -> SquareWaveDetector1/2(CurrentAnalogInOld)
  SquareWaveDetector/1(currentValue) -> Logical Operator/1
  SquareWaveDetector1/1(currentValue) -> Logical Operator/2
  Logical Operator/1 -> current/1

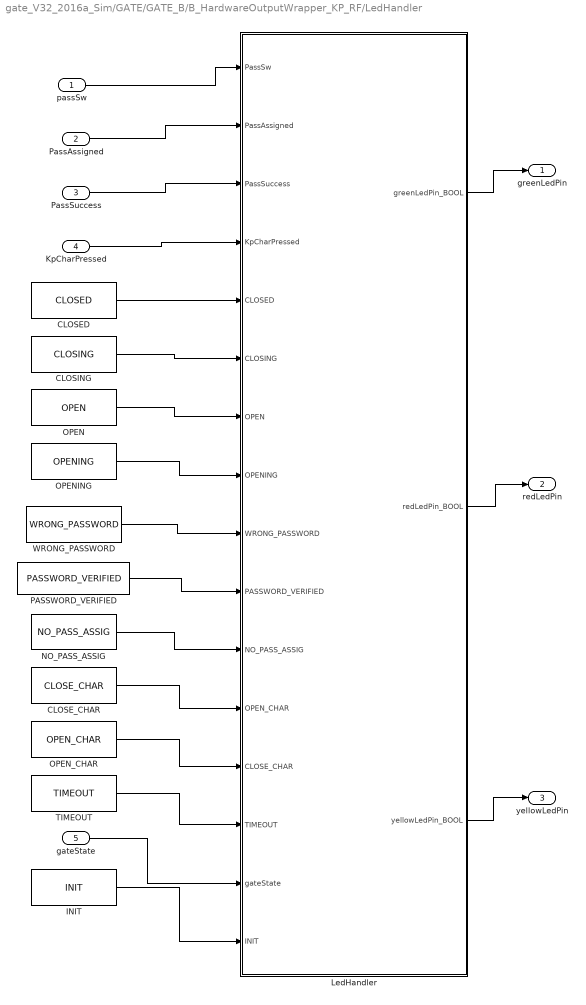
== system gate_V32_2016a_Sim/GATE/GATE_B/B_HardwareOutputWrapper_KP_RF/LedHandler ==
  passSw : Inport
  PassAssigned : Inport  Port=2
  PassSuccess : Inport  Port=3
  KpCharPressed : Inport  Port=4
  gateState : Inport  Port=5
  CLOSED : Constant  Value=CLOSED  SampleTime=-1
  CLOSE_CHAR : Constant  Value=CLOSE_CHAR  SampleTime=-1
  CLOSING : Constant  Value=CLOSING  SampleTime=-1
  INIT : Constant  Value=INIT  SampleTime=-1
  LedHandler : Stateflow chart  TreatAsAtomicUnit=on
  NO_PASS_ASSIG : Constant  Value=NO_PASS_ASSIG  SampleTime=-1
  OPEN : Constant  Value=OPEN  SampleTime=-1
  OPENING : Constant  Value=OPENING  SampleTime=-1
  OPEN_CHAR : Constant  Value=OPEN_CHAR  SampleTime=-1
  PASSWORD_VERIFIED : Constant  Value=PASSWORD_VERIFIED  SampleTime=-1
  TIMEOUT : Constant  Value=TIMEOUT  SampleTime=-1
  WRONG_PASSWORD : Constant  Value=WRONG_PASSWORD  SampleTime=-1
  greenLedPin : Outport
  redLedPin : Outport  Port=2
  yellowLedPin : Outport  Port=3
  wires:
  LedHandler/1(greenLedPin_BOOL) -> greenLedPin/1
  LedHandler/2(redLedPin_BOOL) -> redLedPin/1
  LedHandler/3(yellowLedPin_BOOL) -> yellowLedPin/1
  passSw/1 -> LedHandler/1(PassSw)
  PassAssigned/1 -> LedHandler/2(PassAssigned)
  PassSuccess/1 -> LedHandler/3(PassSuccess)
  OPENING/1 -> LedHandler/8(OPENING)
  OPEN/1 -> LedHandler/7(OPEN)
  CLOSING/1 -> LedHandler/6(CLOSING)
  CLOSED/1 -> LedHandler/5(CLOSED)
  WRONG_PASSWORD/1 -> LedHandler/9(WRONG_PASSWORD)
  PASSWORD_VERIFIED/1 -> LedHandler/10(PASSWORD_VERIFIED)
  NO_PASS_ASSIG/1 -> LedHandler/11(NO_PASS_ASSIG)
  KpCharPressed/1 -> LedHandler/4(KpCharPressed)
  CLOSE_CHAR/1 -> LedHandler/12(OPEN_CHAR)
  OPEN_CHAR/1 -> LedHandler/13(CLOSE_CHAR)
  TIMEOUT/1 -> LedHandler/14(TIMEOUT)
  gateState/1 -> LedHandler/15(gateState)
  INIT/1 -> LedHandler/16(INIT)

== system gate_V32_2016a_Sim/GATE/GATE_B/B_HardwareOutputWrapper_KP_RF/MotorHandler ==
  leftMotor : Inport
  rightMotor : Inport  Port=2
  gateState : Inport  Port=3
  CLOSED : Constant  Value=CLOSED  SampleTime=-1
  CLOSING : Constant  Value=CLOSING  SampleTime=-1
  MotorsHandler : Stateflow chart  TreatAsAtomicUnit=on
  OPEN : Constant  Value=OPEN  SampleTime=-1
  OPENING : Constant  Value=OPENING  SampleTime=-1
  OPENING1 : Constant  Value=INIT  SampleTime=-1
  LeftPin : Outport
  ComPin : Outport  Port=2
  RightPin : Outport  Port=3
  wires:
  rightMotor/1 -> MotorsHandler/2(rightMotor)
  CLOSED/1 -> MotorsHandler/3(CLOSED)
  CLOSING/1 -> MotorsHandler/4(CLOSING)
  OPEN/1 -> MotorsHandler/5(OPEN)
  OPENING/1 -> MotorsHandler/6(OPENING)
  MotorsHandler/1(LeftMotorPin_BOOL) -> LeftPin/1
  MotorsHandler/2(ComMotorPin_BOOL) -> ComPin/1
  MotorsHandler/3(RightMotorPin_BOOL) -> RightPin/1
  gateState/1 -> MotorsHandler/7(gateState)
  leftMotor/1 -> MotorsHandler/1(leftMotor)
  OPENING1/1 -> MotorsHandler/8(INIT)

== system gate_V32_2016a_Sim/GATE/GATE_B/B_HardwareOutputWrapper_KP_RF/SquareWaveCreator ==
  bulbPinIn_BOOL : Inport
  SquareWaveCreator : Stateflow chart  Commented=on  TreatAsAtomicUnit=on
  bulbPin_BOOL : Outport
  wires:
  bulbPinIn_BOOL/1 -> bulbPin_BOOL/1

== system gate_V32_2016a_Sim/GATE/GATE_B/CurrentFilterSubsystem/Subsystem ==
  rightCurrentRaw : Inport
  leftCurrentRaw : Inport  Port=2
  Logical Operator : Logic  Operator=OR  AllPortsSameDT=off  OutDataTypeStr=boolean
  Unit Delay : UnitDelay  SampleTime=-1
  Unit Delay1 : UnitDelay  SampleTime=-1
  WRONG_PASSWORD : Constant  Value=CURRENT_STABLE_TIMER  SampleTime=-1
  WRONG_PASSWORD1 : Constant  Value=CURRENT_STABLE_TIMER  SampleTime=-1
  WRONG_PASSWORD2 : Constant  Value=CURRENT_THRESH  SampleTime=-1
  WRONG_PASSWORD3 : Constant  Value=CURRENT_THRESH  SampleTime=-1
  leftSquareWaveDetector : Stateflow chart  TreatAsAtomicUnit=on
  rightSquareWaveDetector : Stateflow chart  TreatAsAtomicUnit=on
  current : Outport
  wires:
  rightCurrentRaw/1 -> rightSquareWaveDetector/1(CurrentAnalogIn), Unit Delay/1
  Unit Delay/1 -> rightSquareWaveDetector/2(CurrentAnalogInOld)
  leftCurrentRaw/1 -> Unit Delay1/1, leftSquareWaveDetector/1(CurrentAnalogIn)
  Unit Delay1/1 -> leftSquareWaveDetector/2(CurrentAnalogInOld)
  rightSquareWaveDetector/1(currentValue) -> Logical Operator/1
  leftSquareWaveDetector/1(currentValue) -> Logical Operator/2
  Logical Operator/1 -> current/1
  WRONG_PASSWORD/1 -> rightSquareWaveDetector/3(CURRENT_STABLE_TIMER)
  WRONG_PASSWORD1/1 -> leftSquareWaveDetector/3(CURRENT_STABLE_TIMER)
  WRONG_PASSWORD2/1 -> rightSquareWaveDetector/4(CURRENT_THRESH)
  WRONG_PASSWORD3/1 -> leftSquareWaveDetector/4(CURRENT_THRESH)

== system gate_V32_2016a_Sim/GATE/GATE_C/C_HardwareOutputWrapper_RF/MotorHandler ==
  leftMotor : Inport
  rightMotor : Inport  Port=2
  CLOSED : Constant  Value=CLOSED  SampleTime=-1
  CLOSING : Constant  Value=CLOSING  SampleTime=-1
  MotorsHandler : Stateflow chart  TreatAsAtomicUnit=on
  OPEN : Constant  Value=OPEN  SampleTime=-1
  OPENING : Constant  Value=OPENING  SampleTime=-1
  Unit Delay{,1..3} (4 alike) : UnitDelay  SampleTime=-1
  LeftPin : Outport
  ComPin : Outport  Port=2
  RightPin : Outport  Port=3
  wires:
  leftMotor/1 -> Unit Delay/1, MotorsHandler/1(leftMotor)
  rightMotor/1 -> Unit Delay1/1, MotorsHandler/3(rightMotor)
  CLOSED/1 -> MotorsHandler/5(CLOSED)
  CLOSING/1 -> MotorsHandler/6(CLOSING)
  OPEN/1 -> MotorsHandler/7(OPEN)
  OPENING/1 -> MotorsHandler/8(OPENING)
  MotorsHandler/1(LeftMotorPin_BOOL) -> LeftPin/1
  MotorsHandler/2(ComMotorPin_BOOL) -> ComPin/1
  MotorsHandler/3(RightMotorPin_BOOL) -> RightPin/1
  Unit Delay/1 -> Unit Delay2/1
  Unit Delay2/1 -> MotorsHandler/2(oldLeft)
  Unit Delay1/1 -> Unit Delay3/1
  Unit Delay3/1 -> MotorsHandler/4(oldRight)

== system gate_V32_2016a_Sim/GATE/GATE_C/CurrentFilterSubsystem/Subsystem ==
  rightCurrentRaw : Inport
  leftCurrentRaw : Inport  Port=2
  Trigger : TriggerPort  TriggerType=function-call  VariantControl=Variant  PortDimensions=1
      settings: AttributesFormatString=%<StatesWhenEnabling>
  Logical Operator : Logic  Operator=OR  AllPortsSameDT=off  OutDataTypeStr=boolean
  SquareWaveDetector : Stateflow chart  TreatAsAtomicUnit=on
  SquareWaveDetector1 : Stateflow chart  TreatAsAtomicUnit=on
  Unit Delay : UnitDelay  SampleTime=-1
  Unit Delay1 : UnitDelay  SampleTime=-1
  current : Outport
      settings: AttributesFormatString=%<OutputWhenDisabled>
  wires:
  Unit Delay/1 -> SquareWaveDetector/2(CurrentAnalogInOld)
  rightCurrentRaw/1 -> Unit Delay/1, SquareWaveDetector/1(CurrentAnalogIn)
  SquareWaveDetector/1(currentValue) -> Logical Operator/1
  leftCurrentRaw/1 -> Unit Delay1/1, SquareWaveDetector1/1(CurrentAnalogIn)
  Unit Delay1/1 -> SquareWaveDetector1/2(CurrentAnalogInOld)
  SquareWaveDetector1/1(currentValue) -> Logical Operator/2
  Logical Operator/1 -> current/1

== stateflow chart gate_V32_2016a_Sim/GATE/GATE_B/CurrentFilterSubsystem/Subsystem/leftSquareWaveDetector ==
  state Running
    entry:
    counterHigh = 0;
    counterLow= 0;
    currentValue = 1;
    state High
      entry:
      counterLow = 0;
    state Low
      entry:
      counterHigh = 0;
    (default) -> High
    High -> High [order 2] : [CurrentAnalogIn > CURRENT_THRESH]
        | /counterHigh++;
    High -> Low [order 1] : [CurrentAnalogIn < CURRENT_THRESH]
    Low -> High [order 1] : [CurrentAnalogIn > CURRENT_THRESH]
    Low -> Low [order 2] : [CurrentAnalogIn < CURRENT_THRESH]
        | /counterLow++;
  state Stop
    entry:
    currentValue = 0;
    stableCounter = 0;
  (default) -> Stop
  Stop -> Running : [((CurrentAnalogInOld > CURRENT_THRESH)...
      |  && (CurrentAnalogIn < CURRENT_THRESH)) ...
      | || ((CurrentAnalogInOld < CURRENT_THRESH)...
      |  && (CurrentAnalogIn > CURRENT_THRESH))]
  Running -> Stop : [(counterHigh >= CURRENT_STABLE_TIMER)...
      |  || (counterLow >= CURRENT_STABLE_TIMER)]
  data: CurrentAnalogIn input; currentValue output uint8; counterHigh local uint16; counterLow local uint16; stableCounter local uint8; CurrentAnalogInOld input; CURRENT_STABLE_TIMER input; CURRENT_THRESH input

== stateflow chart gate_V32_2016a_Sim/GATE/GATE_A/CurrentFilterSubsystem/10msSmapler ==
  (default) -> (junction 2)
  (junction 2) -> (junction 3) : {counter_1ms++;}
  (junction 3) -> (junction 6) : [counter_1ms == 10]
      | {
      | triggerOn;
      | counter_1ms = 0;
      | }
  data: counter_1ms local double
  events: triggerOn output FUNCTION_CALL_EVENT

== stateflow chart gate_V32_2016a_Sim/GATE/GATE_A/CurrentFilterSubsystem/Subsystem/SquareWaveDetector ==
  state Running
    entry:
    counterHigh = 0;
    counterLow= 0;
    currentValue = 1;
    state High
      entry:
      counterLow = 0;
    state Low
      entry:
      counterHigh = 0;
    (default) -> High
    High -> High [order 2] : [CurrentAnalogIn > 1000]
        | /counterHigh++;
    High -> Low [order 1] : [CurrentAnalogIn < 1000]
    Low -> High [order 1] : [CurrentAnalogIn > 1000]
    Low -> Low [order 2] : [CurrentAnalogIn < 1000]
        | /counterLow++
  state Stop
    entry:
    currentValue = 0;
    stableCounter = 0;
    state PosEdge
    state NegEdge
    (default) -> PosEdge
    PosEdge -> NegEdge : [(CurrentAnalogInOld > 1000)...
        |  && (CurrentAnalogIn < 1000)]...
        | /stableCounter += 1;
    NegEdge -> PosEdge : [(CurrentAnalogInOld < 1000)...
        |  && (CurrentAnalogIn > 1000)]...
        | /stableCounter += 1;
  (default) -> Stop
  Stop -> Running : [(CurrentAnalogInOld != CurrentAnalogIn) && stableCounter > 2]
  Running -> Stop : [(counterHigh >= 50)...
      |  || (counterLow >= 50)]
  data: CurrentAnalogIn input; currentValue output uint8; counterHigh local uint16; counterLow local uint16; stableCounter local uint8; CurrentAnalogInOld input

== stateflow chart gate_V32_2016a_Sim/GATE/GATE_A/CurrentFilterSubsystem/Subsystem/SquareWaveDetector1 ==
  state Running
    entry:
    counterHigh = 0;
    counterLow= 0;
    currentValue = 1;
    state High
      entry:
      counterLow = 0;
    state Low
      entry:
      counterHigh = 0;
    (default) -> High
    High -> High [order 2] : [CurrentAnalogIn > 1000]
        | /counterHigh++;
    High -> Low [order 1] : [CurrentAnalogIn < 1000]
    Low -> High [order 1] : [CurrentAnalogIn > 1000]
    Low -> Low [order 2] : [CurrentAnalogIn < 1000]
        | /counterLow++
  state Stop
    entry:
    currentValue = 0;
    stableCounter = 0;
    state PosEdge
    state NegEdge
    (default) -> PosEdge
    PosEdge -> NegEdge : [(CurrentAnalogInOld > 1000)...
        |  && (CurrentAnalogIn < 1000)]...
        | /stableCounter += 1;
    NegEdge -> PosEdge : [(CurrentAnalogInOld < 1000)...
        |  && (CurrentAnalogIn > 1000)]...
        | /stableCounter += 1;
  (default) -> Stop
  Stop -> Running : [(CurrentAnalogInOld != CurrentAnalogIn) && stableCounter > 2]
  Running -> Stop : [(counterHigh >= 50)...
      |  || (counterLow >= 50)]
  data: CurrentAnalogIn input; currentValue output uint8; counterHigh local uint16; counterLow local uint16; stableCounter local uint8; CurrentAnalogInOld input

== stateflow chart gate_V32_2016a_Sim/GATE/GATE_A/RFHandler/RFHandlerL ==
  state Close
    entry:
    RFOpen = false;
    RFClose = true;
  state RFOff
    entry:
    RFOpen = false;
    RFClose = false;
  state Open
    entry:
    RFOpen = true;
    RFClose = false;
    counter = 0;
    du:
    counter++;
  Close -> RFOff [order 1] : [rightMotor == CLOSED]
  Close -> (junction 11) [order 2] : [hasChanged(btn)]
  (junction 11) -> Close [order 2] : [(btn == 1) ...
      | && ((leftMotor == OPENING)...
      | || (leftMotor == OPEN))]
  (default) -> RFOff
  RFOff -> (junction 11) : [hasChanged(btn)]
  Open -> (junction 11) [order 2] : [hasChanged(btn)]
  (junction 11) -> Open [order 1] : [(btn == 1) ...
      | && ((leftMotor == CLOSING)...
      | || (leftMotor == CLOSED))]
  Open -> RFOff [order 1] : [(counter == 5) ...
      | && ((leftMotor == CLOSING)...
      | || (leftMotor == CLOSED))]
  data: btn input; RFClose output boolean; RFOpen output boolean; leftMotor input; rightMotor input; CLOSED input; CLOSING input; OPEN input; OPENING input; counter local uint8

== stateflow chart gate_V32_2016a_Sim/GATE/GATE_C/CurrentFilterSubsystem/Subsystem/SquareWaveDetector1 ==
  state Running
    entry:
    counterHigh = 0;
    counterLow= 0;
    currentValue = 1;
    state High
      entry:
      counterLow = 0;
    state Low
      entry:
      counterHigh = 0;
    (default) -> High
    High -> High [order 2] : [CurrentAnalogIn > 1000]
        | /counterHigh++;
    High -> Low [order 1] : [CurrentAnalogIn < 1000]
    Low -> High [order 1] : [CurrentAnalogIn > 1000]
    Low -> Low [order 2] : [CurrentAnalogIn < 1000]
        | /counterLow++;
  state Stop
    entry:
    currentValue = 0;
    stableCounter = 0;
    state PosEdge
    state NegEdge
    (default) -> PosEdge
    PosEdge -> NegEdge : [(CurrentAnalogInOld > 1000)...
        |  && (CurrentAnalogIn < 1000)]...
        | /stableCounter += 1;
    NegEdge -> PosEdge : [(CurrentAnalogInOld < 1000)...
        |  && (CurrentAnalogIn > 1000)]...
        | /stableCounter += 1;
  (default) -> Stop
  Stop -> Running : [(CurrentAnalogInOld != CurrentAnalogIn) && stableCounter > 2]
  Running -> Stop : [(counterHigh >= 70)...
      |  || (counterLow >= 70)]
  data: CurrentAnalogIn input; currentValue output uint8; counterHigh local uint16; counterLow local uint16; stableCounter local uint8; CurrentAnalogInOld input

== stateflow chart gate_V32_2016a_Sim/GATE/GATE_B/B_HardwareOutputWrapper_KP_RF/SquareWaveCreator/SquareWaveCreator ==
  state BulbOn
    state Off
      entry:
      counter = 0;
      bulbPin_BOOL = false;
      du:
      counter++;
    state On
      entry:
      counter = 0;
      bulbPin_BOOL = true;
      du:
      counter++;
    (default) -> Off
    On -> Off : [counter >= 1000]/counter = 0;
    Off -> On : [counter >= 1000]/counter = 0;
  state BulbOff
    entry:
    bulbPin_BOOL = false;
  (default) -> BulbOff
  BulbOff -> BulbOn : [bulbPinIn_BOOL_in]
  BulbOn -> BulbOff : [!bulbPinIn_BOOL_in]
  data: bulbPinIn_BOOL_in input; bulbPin_BOOL output boolean; counter local uint16
